simulink subsystem "contactors"  (R2022b)
settings: Solver=VariableStepAuto  StartTime=0.0  StopTime=10.0  RelTol=1e-3
libraries: Raptor_lib x4
settings Model: Creator=serga  LastModifiedBy=serga

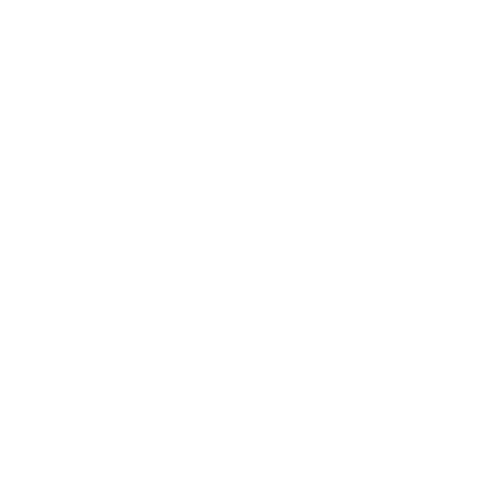
[thumbnail: Simulink's stored preview of the top-level diagram]
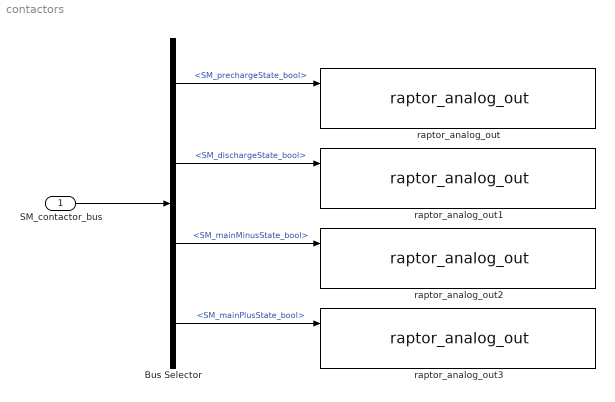
== system contactors ==
  SM_contactor_bus : Inport
  Bus Selector : BusSelector  OutputSignals=SM_prechargeState_bool,SM_dischargeState_bool,SM_mainMinusState_bool,SM_mainPlusState_bool
  raptor_analog_out{,1..3} (4 alike) : Raptor_lib/Input & Output/raptor_analog_out  resourceValues=[]  resource=[]
      settings: SourceProductName=Raptor
  wires:
  SM_contactor_bus/1 -> Bus Selector/1
  Bus Selector/1 -> raptor_analog_out/1  "<SM_prechargeState_bool>"
  Bus Selector/2 -> raptor_analog_out1/1  "<SM_dischargeState_bool>"
  Bus Selector/3 -> raptor_analog_out2/1  "<SM_mainMinusState_bool>"
  Bus Selector/4 -> raptor_analog_out3/1  "<SM_mainPlusState_bool>"
